simulink model "Punto4"  (R2019b)
settings: Solver=VariableStepAuto  StartTime=0.0  StopTime=10.0  RelTol=1e-3
undefined symbols (not defined in the file or in its folder): DiscIntNeverNeededParam
libraries: simulink x1
settings Model: EnablePacing=on  Creator=USER  LastModifiedBy=USER

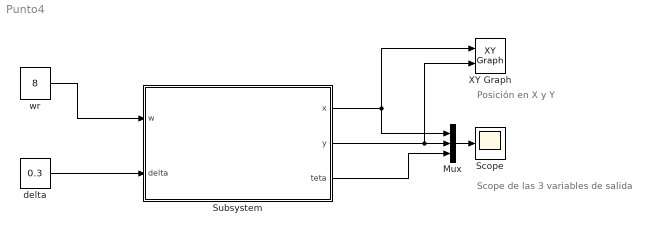
== system Punto4 ==
  note: Posición en X y Y
  note: Scope de las 3 variables de salida
  Mux : Mux  Inputs=3
  Scope : Scope
  Subsystem : Subsystem  mask{WheelRadius=0.5, WheelBase=1.5, Sample_time=0.01, Initial_x=0, Initial_y=0, Initial_t=pi}
      mask prompts: WheelRadius "Wheel Radius"; WheelBase "Wheel_base"; Sample_time "Sample time"; Initial_x "Initial position x"; Initial_y "Inital position y"; Initial_t "Inital Orientation"
  XY Graph : simulink/Sinks/XY Graph  xmin=-10  xmax=10  ymin=-10  ymax=10  st=-1
  delta : Constant  Value=0.3
  wr : Constant  Value=8
  wires:
  Mux/1 -> Scope/1
  wr/1 -> Subsystem/1(w)
  delta/1 -> Subsystem/2(delta)
  Subsystem/1(x) -> XY Graph/1, Mux/1
  Subsystem/2(y) -> XY Graph/2, Mux/2
  Subsystem/3(teta) -> Mux/3

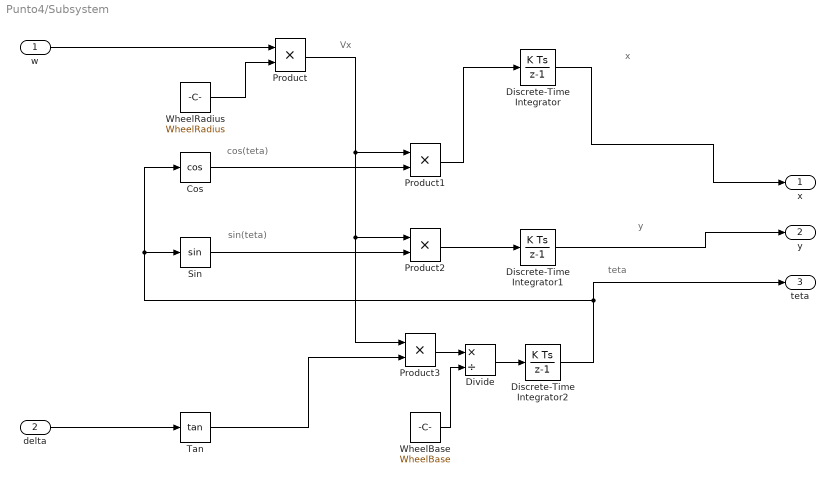
== system Punto4/Subsystem ==
  note: sin(teta)
  note: teta
  note: cos(teta)
  note: Vx
  note: x
  note: y
  w : Inport
  delta : Inport  Port=2
  Cos : Trigonometry  Operator=cos
  Discrete-Time Integrator : DiscreteIntegrator  InitialCondition=Initial_x  SampleTime=Sample_time  ICPrevOutput=DiscIntNeverNeededParam  ICPrevScaledInput=DiscIntNeverNeededParam
  Discrete-Time Integrator1 : DiscreteIntegrator  InitialCondition=Initial_y  SampleTime=Sample_time  ICPrevOutput=DiscIntNeverNeededParam  ICPrevScaledInput=DiscIntNeverNeededParam
  Discrete-Time Integrator2 : DiscreteIntegrator  InitialCondition=Initial_t  SampleTime=Sample_time  ICPrevOutput=DiscIntNeverNeededParam  ICPrevScaledInput=DiscIntNeverNeededParam
  Divide : Product  Inputs=*/
  Product{,1..3} (4 alike) : Product
  Sin : Trigonometry
  Tan : Trigonometry  Operator=tan
  WheelBase : Constant  Value=WheelBase
  WheelRadius : Constant  Value=WheelRadius
  x : Outport
  y : Outport  Port=2
  teta : Outport  Port=3
  wires:
  Sin/1 -> Product2/2
  Product/1 -> Product3/1, Product2/1, Product1/1
  Product3/1 -> Divide/1
  Cos/1 -> Product1/2
  Product1/1 -> Discrete-Time Integrator/1
  Discrete-Time Integrator1/1 -> y/1
  Discrete-Time Integrator2/1 -> teta/1, Sin/1, Cos/1
  Discrete-Time Integrator/1 -> x/1
  Divide/1 -> Discrete-Time Integrator2/1
  WheelBase/1 -> Divide/2
  Tan/1 -> Product3/2
  WheelRadius/1 -> Product/2
  Product2/1 -> Discrete-Time Integrator1/1
  delta/1 -> Tan/1
  w/1 -> Product/1
